simulink model "Lab2_P2Q1d"  (R2019a)
settings: Solver=FixedStepDiscrete  StartTime=0.0  StopTime=10.0  FixedStep=0.01  RelTol=1e-3
settings Model: Creator=keeshigan  LastModifiedBy=keeshigan

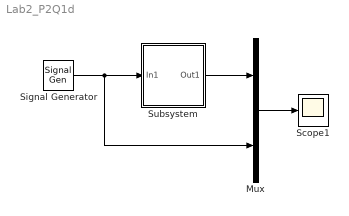
== system Lab2_P2Q1d ==
  Mux : Mux  Inputs=2
  Scope1 : Scope
  Signal Generator : SignalGenerator  WaveForm=square
  Subsystem : Subsystem
  wires:
  Subsystem/1(Out1) -> Mux/1
  Mux/1 -> Scope1/1
  Signal Generator/1 -> Mux/2, Subsystem/1(In1)

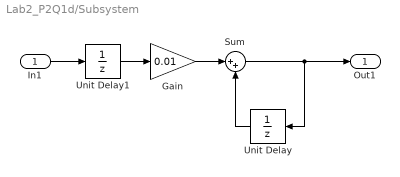
== system Lab2_P2Q1d/Subsystem ==
  In1 : Inport
  Gain : Gain  Gain=0.01
  Sum : Sum  Inputs=|++
  Unit Delay : UnitDelay  SampleTime=-1  HasFrameUpgradeWarning=on
  Unit Delay1 : UnitDelay  SampleTime=-1  HasFrameUpgradeWarning=on
  Out1 : Outport
  wires:
  Unit Delay1/1 -> Gain/1
  Unit Delay/1 -> Sum/2
  In1/1 -> Unit Delay1/1
  Gain/1 -> Sum/1
  Sum/1 -> Out1/1, Unit Delay/1
